simulink model "Final_Project_v3b"  (R2013a)
settings: Solver=ode45  StartTime=0.0  StopTime=inf  RelTol=1e-3
InitFcn:
  | start_EEVSCube2
  | 
  | %links masses
  | 
  | m=20;%Kg
  | 
  | l=1;%meter
  | 
  | %controls
  | 
  | a=0.3; %singularity positive gain
  | 
  | %Chaser
  | 
  | lb=1;%meter distance 1joint to CM
  | 
  | %Target
  | 
  | mt=5;%kg target mass
  | lt=1;%meter  side lenght
  | It=(1/6)*(lt^2);
  | 
  | %Target Initial Conitions
  | 
  | x_t=2;
  | y_t=3;
  | theta_t=0.7853;
  | 
  | Init_t=[x_t;y_t;theta_t];
undefined symbols (not defined in the file or in its folder): mesh_A, mesh_B
libraries: vrlib x2, dspinverses x1, aerolibanimutils x1
(part 2 of 2)

== matlab function Final_Project_v3b/Torque Control/C Matrix ==
  data: qqd input; C output; m parameter; l parameter; q_dot output
function [C,q_dot] = fcn(qqd,m,l)
q=[qqd(7); qqd(8); qqd(9)];
q_dot=[qqd(4); qqd(5); qqd(6)];
C=[                                                                                                                                                                                                                                                                                                                                                                                                                                                                                                                                                  (m*abs(l)^2*(2*sin(conj(q(1))) + sin(conj(q(1)) + conj(q(2)) + conj(q(3))) + 2*sin(conj(q(1)) + conj(q(2))))*(cos(q(1) + q(2) + q(3))*(q_dot(1) + q_dot(2) + q_dot(3)) + 2*cos(q(1) + q(2))*(q_dot(1) + q_dot(2)) + 2*q_dot(1)*cos(q(1))))/8 - (m*abs(l)^2*(2*cos(conj(q(1))) + cos(conj(q(1)) + conj(q(2)) + conj(q(3))) + 2*cos(conj(q(1)) + conj(q(2))))*(sin(q(1) + q(2) + q(3))*(q_dot(1) + q_dot(2) + q_dot(3)) + 2*sin(q(1) + q(2))*(q_dot(1) + q_dot(2)) + 2*q_dot(1)*sin(q(1))))/8 + (m*abs(l)^2*(cos(q(1) + q(2))*(q_dot(1) + q_dot(2)) + 2*q_dot(1)*cos(q(1)))*(2*sin(conj(q(1))) + sin(conj(q(1)) + conj(q(2)))))/8 - (m*abs(l)^2*(2*cos(conj(q(1))) + cos(conj(q(1)) + conj(q(2))))*(sin(q(1) + q(2))*(q_dot(1) + q_dot(2)) + 2*q_dot(1)*sin(q(1))))/8 - (m*abs(l)^2*(cos(q(1) + q(2)) + 2*cos(q(1)))*(2*sin(conj(q(1)))*conj(q_dot(1)) + sin(conj(q(1)) + conj(q(2)))*(conj(q_dot(1)) + conj(q_dot(2)))))/8 + (m*abs(l)^2*(sin(q(1) + q(2)) + 2*sin(q(1)))*(2*cos(conj(q(1)))*conj(q_dot(1)) + cos(conj(q(1)) + conj(q(2)))*(conj(q_dot(1)) + conj(q_dot(2)))))/8 + (m*abs(l)^2*(2*cos(conj(q(1)))*conj(q_dot(1)) + cos(conj(q(1)) + conj(q(2)) + conj(q(3)))*(conj(q_dot(1)) + conj(q_dot(2)) + conj(q_dot(3))) + 2*cos(conj(q(1)) + conj(q(2)))*(conj(q_dot(1)) + conj(q_dot(2))))*(sin(q(1) + q(2) + q(3)) + 2*sin(q(1) + q(2)) + 2*sin(q(1))))/8 - (m*abs(l)^2*(2*sin(conj(q(1)))*conj(q_dot(1)) + sin(conj(q(1)) + conj(q(2)) + conj(q(3)))*(conj(q_dot(1)) + conj(q_dot(2)) + conj(q_dot(3))) + 2*sin(conj(q(1)) + conj(q(2)))*(conj(q_dot(1)) + conj(q_dot(2))))*(cos(q(1) + q(2) + q(3)) + 2*cos(q(1) + q(2)) + 2*cos(q(1))))/8 - (m*q_dot(1)*cos(conj(q(1)))*abs(l)^2*sin(q(1)))/8 + (m*q_dot(1)*sin(conj(q(1)))*abs(l)^2*cos(q(1)))/8 + (m*cos(conj(q(1)))*abs(l)^2*conj(q_dot(1))*sin(q(1)))/8 - (m*sin(conj(q(1)))*abs(l)^2*cos(q(1))*conj(q_dot(1)))/8,                                                                                                                                                                                                                                     (m*sin(conj(q(1)) - q(2) - q(3) - q(1))*abs(l)^2)/2 + (3*m*sin(conj(q(1)) - q(2) - q(1))*abs(l)^2)/4 + (m*abs(l)^2*sin(conj(q(1)) - q(2) - q(3) - q(1) + conj(q(2)))*(q_dot(1) + q_dot(2) + q_dot(3) - conj(q_dot(1)) - conj(q_dot(2))))/4 + (m*sin(conj(q(1)) - q(2) - q(3) - q(1) + conj(q(2)) + conj(q(3)))*abs(l)^2*(q_dot(1) + q_dot(2) + q_dot(3) - conj(q_dot(1)) - conj(q_dot(2)) - conj(q_dot(3))))/8 - (m*sin(q(1) + q(2))*abs(l)^2*(2*cos(conj(q(1))) + cos(conj(q(1)) + conj(q(2)))))/8 + (m*cos(q(1) + q(2))*abs(l)^2*(2*sin(conj(q(1))) + sin(conj(q(1)) + conj(q(2)))))/8 - (m*abs(l)^2*(sin(conj(q(1)) + conj(q(2)) + conj(q(3))) + 2*sin(conj(q(1)) + conj(q(2))))*(cos(q(1) + q(2) + q(3)) + 2*cos(q(1) + q(2)) + 2*cos(q(1))))/8 + (m*abs(l)^2*(cos(conj(q(1)) + conj(q(2)) + conj(q(3))) + 2*cos(conj(q(1)) + conj(q(2))))*(sin(q(1) + q(2) + q(3)) + 2*sin(q(1) + q(2)) + 2*sin(q(1))))/8 - (m*abs(l)^2*sin(conj(q(1)) - q(2) - q(1) + conj(q(2)) + conj(q(3)))*(conj(q_dot(1)) - q_dot(2) - q_dot(1) + conj(q_dot(2)) + conj(q_dot(3))))/4 - (m*abs(l)^2*(sin(q(1) + q(2) + q(3)) + 2*sin(q(1) + q(2)))*(2*cos(conj(q(1))) + cos(conj(q(1)) + conj(q(2)) + conj(q(3))) + 2*cos(conj(q(1)) + conj(q(2)))))/8 + (m*abs(l)^2*(cos(q(1) + q(2) + q(3)) + 2*cos(q(1) + q(2)))*(2*sin(conj(q(1))) + sin(conj(q(1)) + conj(q(2)) + conj(q(3))) + 2*sin(conj(q(1)) + conj(q(2)))))/8 - (m*sin(conj(q(1)) + conj(q(2)))*abs(l)^2*(cos(q(1) + q(2)) + 2*cos(q(1))))/8 + (3*m*sin(conj(q(1)) - q(2) - q(1))*abs(l)^2*(q_dot(1) + q_dot(2) - conj(q_dot(1))))/4 + (m*cos(conj(q(1)) + conj(q(2)))*abs(l)^2*(sin(q(1) + q(2)) + 2*sin(q(1))))/8 + (5*m*sin(conj(q(1)) - q(2) - q(1) + conj(q(2)))*abs(l)^2*(q_dot(1) + q_dot(2) - conj(q_dot(1)) - conj(q_dot(2))))/8 + (m*sin(conj(q(1)) - q(2) - q(3) - q(1))*abs(l)^2*(q_dot(1) + q_dot(2) + q_dot(3) - conj(q_dot(1))))/4, (m*sin(conj(q(1)) - q(2) - q(3) - q(1))*abs(l)^2)/4 + (m*abs(l)^2*(2*sin(conj(q(1)) - q(2) - q(3) - q(1)) + 2*sin(conj(q(1)) - q(2) - q(3) - q(1) + conj(q(2)))))/8 + (m*abs(l)^2*(2*sin(conj(q(1)) - q(2) - q(3) - q(1))*(q_dot(1) + q_dot(2) + q_dot(3) - conj(q_dot(1))) + 2*sin(conj(q(1)) - q(2) - q(3) - q(1) + conj(q(2)))*(q_dot(1) + q_dot(2) + q_dot(3) - conj(q_dot(1)) - conj(q_dot(2))) + sin(conj(q(1)) - q(2) - q(3) - q(1) + conj(q(2)) + conj(q(3)))*(q_dot(1) + q_dot(2) + q_dot(3) - conj(q_dot(1)) - conj(q_dot(2)) - conj(q_dot(3)))))/8 + (m*abs(l)^2*sin(conj(q(1)) - q(2) - q(3) - q(1) + conj(q(2))))/4 - (m*abs(l)^2*sin(conj(q(1)) - q(2) - q(1) + conj(q(2)) + conj(q(3))))/4 + (m*cos(conj(q(1)) + conj(q(2)) + conj(q(3)))*abs(l)^2*(sin(q(1) + q(2) + q(3)) + 2*sin(q(1) + q(2)) + 2*sin(q(1))))/8 - (m*sin(q(1) + q(2) + q(3))*abs(l)^2*(2*cos(conj(q(1))) + cos(conj(q(1)) + conj(q(2)) + conj(q(3))) + 2*cos(conj(q(1)) + conj(q(2)))))/8 + (m*cos(q(1) + q(2) + q(3))*abs(l)^2*(2*sin(conj(q(1))) + sin(conj(q(1)) + conj(q(2)) + conj(q(3))) + 2*sin(conj(q(1)) + conj(q(2)))))/8 - (m*sin(conj(q(1)) + conj(q(2)) + conj(q(3)))*abs(l)^2*(cos(q(1) + q(2) + q(3)) + 2*cos(q(1) + q(2)) + 2*cos(q(1))))/8;
 (m*sin(conj(q(1)) - q(2) - q(3) - q(1))*abs(l)^2)/2 + (3*m*sin(conj(q(1)) - q(2) - q(1))*abs(l)^2)/4 - (m*abs(l)^2*(cos(conj(q(1)) + conj(q(2)) + conj(q(3))) + 2*cos(conj(q(1)) + conj(q(2))))*(sin(q(1) + q(2) + q(3))*(q_dot(1) + q_dot(2) + q_dot(3)) + 2*sin(q(1) + q(2))*(q_dot(1) + q_dot(2)) + 2*q_dot(1)*sin(q(1))))/8 - (m*sin(q(1) + q(2))*abs(l)^2*(2*cos(conj(q(1))) + cos(conj(q(1)) + conj(q(2)))))/8 + (m*cos(q(1) + q(2))*abs(l)^2*(2*sin(conj(q(1))) + sin(conj(q(1)) + conj(q(2)))))/8 - (m*abs(l)^2*(sin(conj(q(1)) + conj(q(2)) + conj(q(3))) + 2*sin(conj(q(1)) + conj(q(2))))*(cos(q(1) + q(2) + q(3)) + 2*cos(q(1) + q(2)) + 2*cos(q(1))))/8 + (m*abs(l)^2*(cos(conj(q(1)) + conj(q(2)) + conj(q(3))) + 2*cos(conj(q(1)) + conj(q(2))))*(sin(q(1) + q(2) + q(3)) + 2*sin(q(1) + q(2)) + 2*sin(q(1))))/8 - (m*abs(l)^2*(sin(conj(q(1)) + conj(q(2)) + conj(q(3)))*(conj(q_dot(1)) + conj(q_dot(2)) + conj(q_dot(3))) + 2*sin(conj(q(1)) + conj(q(2)))*(conj(q_dot(1)) + conj(q_dot(2))))*(cos(q(1) + q(2) + q(3)) + 2*cos(q(1) + q(2)) + 2*cos(q(1))))/8 + (m*abs(l)^2*(cos(conj(q(1)) + conj(q(2)) + conj(q(3)))*(conj(q_dot(1)) + conj(q_dot(2)) + conj(q_dot(3))) + 2*cos(conj(q(1)) + conj(q(2)))*(conj(q_dot(1)) + conj(q_dot(2))))*(sin(q(1) + q(2) + q(3)) + 2*sin(q(1) + q(2)) + 2*sin(q(1))))/8 - (m*abs(l)^2*(sin(q(1) + q(2) + q(3)) + 2*sin(q(1) + q(2)))*(2*cos(conj(q(1))) + cos(conj(q(1)) + conj(q(2)) + conj(q(3))) + 2*cos(conj(q(1)) + conj(q(2)))))/8 + (m*abs(l)^2*(cos(q(1) + q(2) + q(3)) + 2*cos(q(1) + q(2)))*(2*sin(conj(q(1))) + sin(conj(q(1)) + conj(q(2)) + conj(q(3))) + 2*sin(conj(q(1)) + conj(q(2)))))/8 - (m*sin(conj(q(1)) + conj(q(2)))*abs(l)^2*(cos(q(1) + q(2)) + 2*cos(q(1))))/8 + (m*cos(conj(q(1)) + conj(q(2)))*abs(l)^2*(sin(q(1) + q(2)) + 2*sin(q(1))))/8 + (m*sin(conj(q(1)) + conj(q(2)))*abs(l)^2*(cos(q(1) + q(2))*(q_dot(1) + q_dot(2)) + 2*q_dot(1)*cos(q(1))))/8 - (m*cos(conj(q(1)) + conj(q(2)))*abs(l)^2*(sin(q(1) + q(2))*(q_dot(1) + q_dot(2)) + 2*q_dot(1)*sin(q(1))))/8 + (m*abs(l)^2*(sin(conj(q(1)) + conj(q(2)) + conj(q(3))) + 2*sin(conj(q(1)) + conj(q(2))))*(cos(q(1) + q(2) + q(3))*(q_dot(1) + q_dot(2) + q_dot(3)) + 2*cos(q(1) + q(2))*(q_dot(1) + q_dot(2)) + 2*q_dot(1)*cos(q(1))))/8 - (m*sin(conj(q(1)) + conj(q(2)))*abs(l)^2*(conj(q_dot(1)) + conj(q_dot(2)))*(cos(q(1) + q(2)) + 2*cos(q(1))))/8 + (m*cos(conj(q(1)) + conj(q(2)))*abs(l)^2*(conj(q_dot(1)) + conj(q_dot(2)))*(sin(q(1) + q(2)) + 2*sin(q(1))))/8, (m*sin(conj(q(1)) + conj(q(2)))*cos(q(1) + q(2))*abs(l)^2)/4 - (m*cos(conj(q(1)) + conj(q(2)))*sin(q(1) + q(2))*abs(l)^2)/4 - (m*abs(l)^2*(sin(conj(q(1)) + conj(q(2)) + conj(q(3))) + 2*sin(conj(q(1)) + conj(q(2))))*(cos(q(1) + q(2) + q(3)) + 2*cos(q(1) + q(2)) + 2*cos(q(1))))/4 + (m*abs(l)^2*(cos(conj(q(1)) + conj(q(2)) + conj(q(3))) + 2*cos(conj(q(1)) + conj(q(2))))*(sin(q(1) + q(2) + q(3)) + 2*sin(q(1) + q(2)) + 2*sin(q(1))))/4 - (m*abs(l)^2*(cos(q(1) + q(2) + q(3)) + 2*cos(q(1) + q(2)))*(sin(conj(q(1)) + conj(q(2)) + conj(q(3)))*(conj(q_dot(1)) + conj(q_dot(2)) + conj(q_dot(3))) + 2*sin(conj(q(1)) + conj(q(2)))*(conj(q_dot(1)) + conj(q_dot(2)))))/8 + (m*abs(l)^2*(sin(q(1) + q(2) + q(3)) + 2*sin(q(1) + q(2)))*(cos(conj(q(1)) + conj(q(2)) + conj(q(3)))*(conj(q_dot(1)) + conj(q_dot(2)) + conj(q_dot(3))) + 2*cos(conj(q(1)) + conj(q(2)))*(conj(q_dot(1)) + conj(q_dot(2)))))/8 - (m*abs(l)^2*(cos(conj(q(1)) + conj(q(2)) + conj(q(3))) + 2*cos(conj(q(1)) + conj(q(2))))*(sin(q(1) + q(2) + q(3))*(q_dot(1) + q_dot(2) + q_dot(3)) + 2*sin(q(1) + q(2))*(q_dot(1) + q_dot(2))))/8 + (m*abs(l)^2*(sin(conj(q(1)) + conj(q(2)) + conj(q(3))) + 2*sin(conj(q(1)) + conj(q(2))))*(cos(q(1) + q(2) + q(3))*(q_dot(1) + q_dot(2) + q_dot(3)) + 2*cos(q(1) + q(2))*(q_dot(1) + q_dot(2))))/8 - (m*sin(conj(q(1)) + conj(q(2)))*abs(l)^2*(cos(q(1) + q(2)) + 2*cos(q(1))))/4 + (m*cos(conj(q(1)) + conj(q(2)))*abs(l)^2*(sin(q(1) + q(2)) + 2*sin(q(1))))/4 - (m*abs(l)^2*(cos(conj(q(1)) + conj(q(2)) + conj(q(3))) + 2*cos(conj(q(1)) + conj(q(2))))*(sin(q(1) + q(2) + q(3)) + 2*sin(q(1) + q(2))))/4 + (m*abs(l)^2*(cos(q(1) + q(2) + q(3)) + 2*cos(q(1) + q(2)))*(sin(conj(q(1)) + conj(q(2)) + conj(q(3))) + 2*sin(conj(q(1)) + conj(q(2)))))/4 + (m*cos(conj(q(1)) + conj(q(2)))*sin(q(1) + q(2))*abs(l)^2*(conj(q_dot(1)) + conj(q_dot(2))))/8 - (m*sin(conj(q(1)) + conj(q(2)))*cos(q(1) + q(2))*abs(l)^2*(conj(q_dot(1)) + conj(q_dot(2))))/8 - (m*cos(conj(q(1)) + conj(q(2)))*sin(q(1) + q(2))*abs(l)^2*(q_dot(1) + q_dot(2)))/8 + (m*sin(conj(q(1)) + conj(q(2)))*cos(q(1) + q(2))*abs(l)^2*(q_dot(1) + q_dot(2)))/8,                                                                                                                                                                                                                                                                                                                       (m*abs(l)^2*(2*sin(conj(q(1)) - q(2) - q(3) - q(1) + conj(q(2)))*(q_dot(1) + q_dot(2) + q_dot(3) - conj(q_dot(1)) - conj(q_dot(2))) + sin(conj(q(1)) - q(2) - q(3) - q(1) + conj(q(2)) + conj(q(3)))*(q_dot(1) + q_dot(2) + q_dot(3) - conj(q_dot(1)) - conj(q_dot(2)) - conj(q_dot(3)))))/8 + (m*abs(l)^2*sin(conj(q(1)) - q(2) - q(3) - q(1) + conj(q(2))))/4 + (m*cos(conj(q(1)) + conj(q(2)) + conj(q(3)))*abs(l)^2*(sin(q(1) + q(2) + q(3)) + 2*sin(q(1) + q(2)) + 2*sin(q(1))))/4 - (m*sin(q(1) + q(2) + q(3))*abs(l)^2*(cos(conj(q(1)) + conj(q(2)) + conj(q(3))) + 2*cos(conj(q(1)) + conj(q(2)))))/4 + (m*cos(q(1) + q(2) + q(3))*abs(l)^2*(sin(conj(q(1)) + conj(q(2)) + conj(q(3))) + 2*sin(conj(q(1)) + conj(q(2)))))/4 - (m*sin(conj(q(1)) + conj(q(2)) + conj(q(3)))*abs(l)^2*(cos(q(1) + q(2) + q(3)) + 2*cos(q(1) + q(2)) + 2*cos(q(1))))/4;
                                                                                                                                                                                                                                                                                                                                                                                                                                                                                                                                                                                                                                                                                                                                                                                                      (m*sin(conj(q(1)) - q(2) - q(3) - q(1))*abs(l)^2)/4 + (m*abs(l)^2*(2*sin(conj(q(1)) - q(2) - q(3) - q(1)) + 2*sin(conj(q(1)) - q(2) - q(3) - q(1) + conj(q(2)))))/8 + (m*abs(l)^2*sin(conj(q(1)) - q(2) - q(3) - q(1) + conj(q(2))))/4 - (m*abs(l)^2*sin(conj(q(1)) - q(2) - q(1) + conj(q(2)) + conj(q(3))))/4 + (m*cos(conj(q(1)) + conj(q(2)) + conj(q(3)))*abs(l)^2*(sin(q(1) + q(2) + q(3)) + 2*sin(q(1) + q(2)) + 2*sin(q(1))))/8 - (m*sin(q(1) + q(2) + q(3))*abs(l)^2*(2*cos(conj(q(1))) + cos(conj(q(1)) + conj(q(2)) + conj(q(3))) + 2*cos(conj(q(1)) + conj(q(2)))))/8 + (m*cos(q(1) + q(2) + q(3))*abs(l)^2*(2*sin(conj(q(1))) + sin(conj(q(1)) + conj(q(2)) + conj(q(3))) + 2*sin(conj(q(1)) + conj(q(2)))))/8 + (m*sin(conj(q(1)) + conj(q(2)) + conj(q(3)))*abs(l)^2*(cos(q(1) + q(2) + q(3))*(q_dot(1) + q_dot(2) + q_dot(3)) + 2*cos(q(1) + q(2))*(q_dot(1) + q_dot(2)) + 2*q_dot(1)*cos(q(1))))/8 - (m*cos(conj(q(1)) + conj(q(2)) + conj(q(3)))*abs(l)^2*(sin(q(1) + q(2) + q(3))*(q_dot(1) + q_dot(2) + q_dot(3)) + 2*sin(q(1) + q(2))*(q_dot(1) + q_dot(2)) + 2*q_dot(1)*sin(q(1))))/8 - (m*sin(conj(q(1)) + conj(q(2)) + conj(q(3)))*abs(l)^2*(cos(q(1) + q(2) + q(3)) + 2*cos(q(1) + q(2)) + 2*cos(q(1))))/8 - (m*sin(conj(q(1)) + conj(q(2)) + conj(q(3)))*abs(l)^2*(cos(q(1) + q(2) + q(3)) + 2*cos(q(1) + q(2)) + 2*cos(q(1)))*(conj(q_dot(1)) + conj(q_dot(2)) + conj(q_dot(3))))/8 + (m*cos(conj(q(1)) + conj(q(2)) + conj(q(3)))*abs(l)^2*(sin(q(1) + q(2) + q(3)) + 2*sin(q(1) + q(2)) + 2*sin(q(1)))*(conj(q_dot(1)) + conj(q_dot(2)) + conj(q_dot(3))))/8,                                                                                                                                                                                                                                                                                                                                                                                                                                                                                                                                                                                                                                                                                                                                                                                                            (m*abs(l)^2*sin(conj(q(1)) - q(2) - q(3) - q(1) + conj(q(2))))/4 + (m*cos(conj(q(1)) + conj(q(2)) + conj(q(3)))*abs(l)^2*(sin(q(1) + q(2) + q(3)) + 2*sin(q(1) + q(2)) + 2*sin(q(1))))/4 + (m*sin(conj(q(1)) + conj(q(2)) + conj(q(3)))*abs(l)^2*(cos(q(1) + q(2) + q(3))*(q_dot(1) + q_dot(2) + q_dot(3)) + 2*cos(q(1) + q(2))*(q_dot(1) + q_dot(2))))/8 - (m*cos(conj(q(1)) + conj(q(2)) + conj(q(3)))*abs(l)^2*(sin(q(1) + q(2) + q(3))*(q_dot(1) + q_dot(2) + q_dot(3)) + 2*sin(q(1) + q(2))*(q_dot(1) + q_dot(2))))/8 - (m*sin(q(1) + q(2) + q(3))*abs(l)^2*(cos(conj(q(1)) + conj(q(2)) + conj(q(3))) + 2*cos(conj(q(1)) + conj(q(2)))))/4 + (m*cos(q(1) + q(2) + q(3))*abs(l)^2*(sin(conj(q(1)) + conj(q(2)) + conj(q(3))) + 2*sin(conj(q(1)) + conj(q(2)))))/4 - (m*sin(conj(q(1)) + conj(q(2)) + conj(q(3)))*abs(l)^2*(cos(q(1) + q(2) + q(3)) + 2*cos(q(1) + q(2)) + 2*cos(q(1))))/4 - (m*sin(conj(q(1)) + conj(q(2)) + conj(q(3)))*abs(l)^2*(cos(q(1) + q(2) + q(3)) + 2*cos(q(1) + q(2)))*(conj(q_dot(1)) + conj(q_dot(2)) + conj(q_dot(3))))/8 + (m*cos(conj(q(1)) + conj(q(2)) + conj(q(3)))*abs(l)^2*(sin(q(1) + q(2) + q(3)) + 2*sin(q(1) + q(2)))*(conj(q_dot(1)) + conj(q_dot(2)) + conj(q_dot(3))))/8,                                                                                                                                                                                                                                                                                                                                                            (m*sin(conj(q(1)) - q(2) - q(3) - q(1) + conj(q(2)) + conj(q(3)))*abs(l)^2*(q_dot(1) + q_dot(2) + q_dot(3) - conj(q_dot(1)) - conj(q_dot(2)) - conj(q_dot(3))))/8 + (m*cos(conj(q(1)) + conj(q(2)) + conj(q(3)))*abs(l)^2*(sin(q(1) + q(2) + q(3)) + 2*sin(q(1) + q(2)) + 2*sin(q(1))))/4 + (m*cos(q(1) + q(2) + q(3))*sin(conj(q(1)) + conj(q(2)) + conj(q(3)))*abs(l)^2)/2 - (m*sin(q(1) + q(2) + q(3))*cos(conj(q(1)) + conj(q(2)) + conj(q(3)))*abs(l)^2)/2 - (m*sin(conj(q(1)) + conj(q(2)) + conj(q(3)))*abs(l)^2*(cos(q(1) + q(2) + q(3)) + 2*cos(q(1) + q(2))))/4 + (m*cos(conj(q(1)) + conj(q(2)) + conj(q(3)))*abs(l)^2*(sin(q(1) + q(2) + q(3)) + 2*sin(q(1) + q(2))))/4 - (m*sin(conj(q(1)) + conj(q(2)) + conj(q(3)))*abs(l)^2*(cos(q(1) + q(2) + q(3)) + 2*cos(q(1) + q(2)) + 2*cos(q(1))))/4];

== matlab function Final_Project_v3b/Torque Control/G Matrix (set zero) ==
  data: qqd input; G output; l parameter; m parameter
function G = fcn(qqd,l,m)

q=[qqd(7); qqd(8); qqd(9)];

g=[0 9.81 0]; %gravity acceleration along y


Jp1=[-(l/2)*sin(q(1)) 0 0; (l/2)*cos(q(1)) 0 0; 0 0 0];
Jo1=[0 0 0; 0 0 0; 1 0 0];

Jp2=[-l*sin(q(1))-(l/2)*sin(q(1)+q(2)) -(l/2)*sin(q(1)+q(2)) 0 ;    l*cos(q(1))+(l/2)*cos(q(1)+q(2)) (l/2)*cos(q(1)+q(2)) 0; 0 0 0];
Jo2=[0 0 0; 0 0 0; 1 1 0];

Jp3=[-l*sin(q(1))-l*sin(q(1)+q(2))-(l/2)*sin(q(1)+q(2)+q(3)) -l*sin(q(1)+q(2))-(l/2)*sin(q(1)+q(2)+q(3)) -(l/2)*sin(q(1)+q(2)+q(3)); l*cos(q(1))+(l)*cos(q(1)+q(2))+(l/2)*cos(q(1)+q(2)+q(3)) l*cos(q(1)+q(2))+(l/2)*cos(q(1)+q(2)+q(3)) (l/2)*cos(q(1)+q(2)+q(3)); 0 0 0];
Jo3=[0 0 0; 0 0 0; 1 1 1];

G1=m*(g)*Jp1+m*(g)*Jp2+m*(g)*Jp3;

%G=G1.';

G=[0;0;0];

== matlab function Final_Project_v3b/Torque Control/H Matrix ==
  data: H output; qqd input; l parameter; m parameter
function H = fcn(qqd,l,m)

q=[qqd(7); qqd(8); qqd(9)];
I=(1/12)*m*(l^2); 
%Hand derivation of the Jacobians for the three links
Jp1=[-(l/2)*sin(q(1)) 0 0; (l/2)*cos(q(1)) 0 0; 0 0 0];
Jo1=[0 0 0; 0 0 0; 1 0 0];

Jp2=[-l*sin(q(1))-(l/2)*sin(q(1)+q(2)) -(l/2)*sin(q(1)+q(2)) 0 ;    l*cos(q(1))+(l/2)*cos(q(1)+q(2)) (l/2)*cos(q(1)+q(2)) 0; 0 0 0];
Jo2=[0 0 0; 0 0 0; 1 1 0];

Jp3=[-l*sin(q(1))-l*sin(q(1)+q(2))-(l/2)*sin(q(1)+q(2)+q(3)) -l*sin(q(1)+q(2))-(l/2)*sin(q(1)+q(2)+q(3)) -(l/2)*sin(q(1)+q(2)+q(3)); l*cos(q(1))+(l)*cos(q(1)+q(2))+(l/2)*cos(q(1)+q(2)+q(3)) l*cos(q(1)+q(2))+(l/2)*cos(q(1)+q(2)+q(3)) (l/2)*cos(q(1)+q(2)+q(3)); 0 0 0];
Jo3=[0 0 0; 0 0 0; 1 1 1];

%%%%%%%%%%%%%%%%%%%%%%%%%%%%%%%%%%%%%%%%%%%%%%%%%%%%%%%%%%%%%%%%%%%%%%%%%
% %Inertia Matrix H
H1=(m*(Jp1')*Jp1)+(Jo1'*I*Jo1); %should be Hermitian? ???????????    
H2=(m*(Jp2')*Jp2)+(Jo2'*I*Jo2);
H3=(m*(Jp3')*Jp3)+(Jo3'*I*Jo3);
%Total Inertia Matrix
H=H1+H2+H3;

== matlab function Final_Project_v3b/Dynamics Block/H Matrix ==
  data: H output; qqd input; l parameter; m parameter
function H = fcn(qqd,l,m)

q=[qqd(7) qqd(8) qqd(9)];
I=(1/12)*m*(l^2); 
%Hand derivation of the Jacobians for the three links
Jp1=[-(l/2)*sin(q(1)) 0 0; (l/2)*cos(q(1)) 0 0; 0 0 0];
Jo1=[0 0 0; 0 0 0; 1 0 0];

Jp2=[-l*sin(q(1))-(l/2)*sin(q(1)+q(2)) -(l/2)*sin(q(1)+q(2)) 0 ;    l*cos(q(1))+(l/2)*cos(q(1)+q(2)) (l/2)*cos(q(1)+q(2)) 0; 0 0 0];
Jo2=[0 0 0; 0 0 0; 1 1 0];

Jp3=[-l*sin(q(1))-l*sin(q(1)+q(2))-(l/2)*sin(q(1)+q(2)+q(3)) -l*sin(q(1)+q(2))-(l/2)*sin(q(1)+q(2)+q(3)) -(l/2)*sin(q(1)+q(2)+q(3)); l*cos(q(1))+(l)*cos(q(1)+q(2))+(l/2)*cos(q(1)+q(2)+q(3)) l*cos(q(1)+q(2))+(l/2)*cos(q(1)+q(2)+q(3)) (l/2)*cos(q(1)+q(2)+q(3)); 0 0 0];
Jo3=[0 0 0; 0 0 0; 1 1 1];

%%%%%%%%%%%%%%%%%%%%%%%%%%%%%%%%%%%%%%%%%%%%%%%%%%%%%%%%%%%%%%%%%%%%%%%%%
% %Inertia Matrix H
H1=(m*(Jp1')*Jp1)+(Jo1'*I*Jo1); %should be Hermitian? ???????????    
H2=(m*(Jp2')*Jp2)+(Jo2'*I*Jo2);
H3=(m*(Jp3')*Jp3)+(Jo3'*I*Jo3);
%Total Inertia Matrix
H=H1+H2+H3;

== matlab function Final_Project_v3b/Singularity Check ==
  data: qqd input; Ya output; l parameter
function Ya   = fcn( qqd,l)
%Singularity trigger, Alessio Grompone 2013

q=[qqd(7) qqd(8) qqd(9)];

%if A==0
%Jacobian position only

Ja=[-(l*sin(q(1))+l*sin(q(1)+q(2))+l*sin(q(1)+q(2)+q(3))) -(l*sin(q(1)+q(2))+l*sin(q(1)+q(2)+q(3))) -l*sin(q(1)+q(2)+q(3));
l*cos(q(1))+l*cos(q(1)+q(2))+l*cos(q(1)+q(2)+q(3)) l*cos(q(1)+q(2))+l*cos(q(1)+q(2)+q(3)) l*cos(q(1)+q(2)+q(3))];

Ra=rank(Ja); %rank of the Jacobian
Sa=size(Ja); %dimension of the Jacobian matrix

if Ra<Sa(1)

Ya=0; %non singular

else
    
Ya=1;
    
end

== matlab function Final_Project_v3b/Differential Kinematics/Differential Kinematics and singularity avoidance ==
  data: Ve input; qqd input; qd_req output; qd_reqW output; l parameter; a parameter; W output; EE input
function [qd_req,qd_reqW,W]   = fcn( Ve,qqd, l, a,EE)
%Singularity trigger, Alessio Grompone 2013

%computes the Jacobian of a redundant 3R manipulator (end-effector position
%only)measures the rank and gives an error if the rank is < than the number of
%variables

q=[qqd(7) qqd(8) qqd(9)];

%Jacobian position only

Ja=[-(l*sin(q(1))+l*sin(q(1)+q(2))+l*sin(q(1)+q(2)+q(3))) -(l*sin(q(1)+q(2))+l*sin(q(1)+q(2)+q(3))) -l*sin(q(1)+q(2)+q(3));
l*cos(q(1))+l*cos(q(1)+q(2))+l*cos(q(1)+q(2)+q(3)) l*cos(q(1)+q(2))+l*cos(q(1)+q(2)+q(3)) l*cos(q(1)+q(2)+q(3))];

DDD=det(Ja*Ja');
%     %Singularity Measure
% 
W=sqrt(DDD);
if q(2)==0
    
    DW=[0;0;0];
else
%Derivative of the singularity measure obtained in symbolic form
    DW=[                                                                                                                                                                                                                                                                                                                                                                                                                                                                                                                                                                                                                                                                                                                                                                                                                                                                                                                                                                                                                                                                                                                                                                                                                                                                                                                                                                                                                                                                                                                                                                                                                                                                                                                                                                                                                                                                                                                                                                                                                                                                                                                                                                                                                                                                                                                                                                                                                                                                                                                                                                                                                                                                                                                                                                                                                                                                                                                                                                                                                                                                                                                                                                                                                                                                                                                                                                                                                                                                                                                                                                                                                                                                                                                                                                                                                                                                                                                                                                                                                                                                                                                                                                                                                                                                                                                                                                                                                                                                                                                                                                                                                                                                                                                                                                                                                                                                                                                                                                                                                                                                                                                                                                                                                                                                                                                                                                                                                                                                                                                                                                                                                                                                                                                                                                                  0;
                                                                                                                                                                                                                                                                                                                                                                                                                 -(cos(q(1) + q(2) + q(3))*cos(conj(q(1)) + conj(q(2)) + conj(q(3)))*sin(conj(q(1)) + conj(q(2)))*cos(q(1)) - cos(q(1) + q(2) + q(3))*sin(conj(q(1)) + conj(q(2)) + conj(q(3)))*cos(conj(q(1)) + conj(q(2)))*cos(q(1)) + cos(q(1) + q(2) + q(3))*sin(conj(q(1)))*sin(conj(q(1)) + conj(q(2)))*sin(q(1)) - sin(q(1) + q(2) + q(3))*cos(conj(q(1)))*sin(conj(q(1)) + conj(q(2)))*sin(q(1)) + sin(q(1) + q(2) + q(3))*sin(conj(q(1)))*cos(conj(q(1)) + conj(q(2)))*sin(q(1)) - sin(q(1) + q(2) + q(3))*sin(conj(q(1)))*sin(conj(q(1)) + conj(q(2)))*cos(q(1)) + sin(q(1) + q(2) + q(3))*cos(conj(q(1)) + conj(q(2)) + conj(q(3)))*sin(conj(q(1)) + conj(q(2)))*sin(q(1)) - sin(q(1) + q(2) + q(3))*sin(conj(q(1)) + conj(q(2)) + conj(q(3)))*cos(conj(q(1)) + conj(q(2)))*sin(q(1)) + cos(conj(q(1)))*cos(conj(q(1)) + conj(q(2)) + conj(q(3)))*cos(q(1) + q(2))*sin(q(1)) - cos(conj(q(1)))*cos(conj(q(1)) + conj(q(2)) + conj(q(3)))*sin(q(1) + q(2))*cos(q(1)) - cos(conj(q(1)))*sin(conj(q(1)) + conj(q(2)) + conj(q(3)))*cos(q(1) + q(2))*cos(q(1)) + cos(conj(q(1)) + conj(q(2)) + conj(q(3)))*sin(conj(q(1)))*cos(q(1) + q(2))*cos(q(1)) - cos(conj(q(1)))*sin(conj(q(1)) + conj(q(2)) + conj(q(3)))*sin(q(1) + q(2))*sin(q(1)) + cos(conj(q(1)) + conj(q(2)) + conj(q(3)))*sin(conj(q(1)))*sin(q(1) + q(2))*sin(q(1)) + sin(conj(q(1)))*sin(conj(q(1)) + conj(q(2)) + conj(q(3)))*cos(q(1) + q(2))*sin(q(1)) - sin(conj(q(1)))*sin(conj(q(1)) + conj(q(2)) + conj(q(3)))*sin(q(1) + q(2))*cos(q(1)) + cos(conj(q(1)))*cos(conj(q(1)) + conj(q(2)))*cos(q(1) + q(2))*sin(q(1)) - cos(conj(q(1)))*cos(conj(q(1)) + conj(q(2)))*sin(q(1) + q(2))*cos(q(1)) - cos(conj(q(1)))*sin(conj(q(1)) + conj(q(2)))*cos(q(1) + q(2))*cos(q(1)) + sin(conj(q(1)))*cos(conj(q(1)) + conj(q(2)))*cos(q(1) + q(2))*cos(q(1)) + cos(q(1) + q(2) + q(3))*cos(conj(q(1)))*cos(conj(q(1)) + conj(q(2)) + conj(q(3)))*sin(q(1) + q(2)) - sin(q(1) + q(2) + q(3))*cos(conj(q(1)))*cos(conj(q(1)) + conj(q(2)) + conj(q(3)))*cos(q(1) + q(2)) - cos(conj(q(1)))*sin(conj(q(1)) + conj(q(2)))*sin(q(1) + q(2))*sin(q(1)) + sin(conj(q(1)))*cos(conj(q(1)) + conj(q(2)))*sin(q(1) + q(2))*sin(q(1)) + sin(conj(q(1)))*sin(conj(q(1)) + conj(q(2)))*cos(q(1) + q(2))*sin(q(1)) - sin(conj(q(1)))*sin(conj(q(1)) + conj(q(2)))*sin(q(1) + q(2))*cos(q(1)) + cos(q(1) + q(2) + q(3))*sin(conj(q(1)))*sin(conj(q(1)) + conj(q(2)) + conj(q(3)))*sin(q(1) + q(2)) - sin(q(1) + q(2) + q(3))*sin(conj(q(1)))*sin(conj(q(1)) + conj(q(2)) + conj(q(3)))*cos(q(1) + q(2)) + 2*cos(q(1) + q(2) + q(3))*cos(conj(q(1)))*cos(conj(q(1)) + conj(q(2)) + conj(q(3)))*sin(q(1)) - 2*cos(q(1) + q(2) + q(3))*cos(conj(q(1)))*sin(conj(q(1)) + conj(q(2)) + conj(q(3)))*cos(q(1)) + 2*cos(q(1) + q(2) + q(3))*cos(conj(q(1)) + conj(q(2)) + conj(q(3)))*sin(conj(q(1)))*cos(q(1)) - 2*sin(q(1) + q(2) + q(3))*cos(conj(q(1)))*cos(conj(q(1)) + conj(q(2)) + conj(q(3)))*cos(q(1)) + 2*cos(q(1) + q(2) + q(3))*sin(conj(q(1)))*sin(conj(q(1)) + conj(q(2)) + conj(q(3)))*sin(q(1)) - 2*sin(q(1) + q(2) + q(3))*cos(conj(q(1)))*sin(conj(q(1)) + conj(q(2)) + conj(q(3)))*sin(q(1)) + 2*sin(q(1) + q(2) + q(3))*cos(conj(q(1)) + conj(q(2)) + conj(q(3)))*sin(conj(q(1)))*sin(q(1)) - 2*sin(q(1) + q(2) + q(3))*sin(conj(q(1)))*sin(conj(q(1)) + conj(q(2)) + conj(q(3)))*cos(q(1)) + cos(q(1) + q(2) + q(3))*cos(conj(q(1)))*cos(conj(q(1)) + conj(q(2)))*sin(q(1)) - cos(q(1) + q(2) + q(3))*cos(conj(q(1)))*sin(conj(q(1)) + conj(q(2)))*cos(q(1)) + cos(q(1) + q(2) + q(3))*sin(conj(q(1)))*cos(conj(q(1)) + conj(q(2)))*cos(q(1)) - sin(q(1) + q(2) + q(3))*cos(conj(q(1)))*cos(conj(q(1)) + conj(q(2)))*cos(q(1)))/(2*(cos(q(1) + q(2) + q(3))*sin(conj(q(1)))*cos(conj(q(1)) + conj(q(2)))*sin(q(1)) - cos(q(1) + q(2) + q(3))*cos(conj(q(1)))*sin(conj(q(1)) + conj(q(2)))*sin(q(1)) + sin(q(1) + q(2) + q(3))*cos(conj(q(1)))*sin(conj(q(1)) + conj(q(2)))*cos(q(1)) - sin(q(1) + q(2) + q(3))*sin(conj(q(1)))*cos(conj(q(1)) + conj(q(2)))*cos(q(1)) + cos(q(1) + q(2) + q(3))*cos(conj(q(1)) + conj(q(2)) + conj(q(3)))*sin(conj(q(1)) + conj(q(2)))*sin(q(1)) - cos(q(1) + q(2) + q(3))*sin(conj(q(1)) + conj(q(2)) + conj(q(3)))*cos(conj(q(1)) + conj(q(2)))*sin(q(1)) - sin(q(1) + q(2) + q(3))*cos(conj(q(1)) + conj(q(2)) + conj(q(3)))*sin(conj(q(1)) + conj(q(2)))*cos(q(1)) + sin(q(1) + q(2) + q(3))*sin(conj(q(1)) + conj(q(2)) + conj(q(3)))*cos(conj(q(1)) + conj(q(2)))*cos(q(1)) - cos(conj(q(1)))*sin(conj(q(1)) + conj(q(2)) + conj(q(3)))*cos(q(1) + q(2))*sin(q(1)) + cos(conj(q(1)))*sin(conj(q(1)) + conj(q(2)) + conj(q(3)))*sin(q(1) + q(2))*cos(q(1)) + cos(conj(q(1)) + conj(q(2)) + conj(q(3)))*sin(conj(q(1)))*cos(q(1) + q(2))*sin(q(1)) - cos(conj(q(1)) + conj(q(2)) + conj(q(3)))*sin(conj(q(1)))*sin(q(1) + q(2))*cos(q(1)) - cos(conj(q(1)))*sin(conj(q(1)) + conj(q(2)))*cos(q(1) + q(2))*sin(q(1)) + cos(conj(q(1)))*sin(conj(q(1)) + conj(q(2)))*sin(q(1) + q(2))*cos(q(1)) + sin(conj(q(1)))*cos(conj(q(1)) + conj(q(2)))*cos(q(1) + q(2))*sin(q(1)) - sin(conj(q(1)))*cos(conj(q(1)) + conj(q(2)))*sin(q(1) + q(2))*cos(q(1)) - cos(q(1) + q(2) + q(3))*cos(conj(q(1)))*sin(conj(q(1)) + conj(q(2)) + conj(q(3)))*sin(q(1) + q(2)) + cos(q(1) + q(2) + q(3))*cos(conj(q(1)) + conj(q(2)) + conj(q(3)))*sin(conj(q(1)))*sin(q(1) + q(2)) + sin(q(1) + q(2) + q(3))*cos(conj(q(1)))*sin(conj(q(1)) + conj(q(2)) + conj(q(3)))*cos(q(1) + q(2)) - sin(q(1) + q(2) + q(3))*cos(conj(q(1)) + conj(q(2)) + conj(q(3)))*sin(conj(q(1)))*cos(q(1) + q(2)) - 2*cos(q(1) + q(2) + q(3))*cos(conj(q(1)))*sin(conj(q(1)) + conj(q(2)) + conj(q(3)))*sin(q(1)) + 2*cos(q(1) + q(2) + q(3))*cos(conj(q(1)) + conj(q(2)) + conj(q(3)))*sin(conj(q(1)))*sin(q(1)) + 2*sin(q(1) + q(2) + q(3))*cos(conj(q(1)))*sin(conj(q(1)) + conj(q(2)) + conj(q(3)))*cos(q(1)) - 2*sin(q(1) + q(2) + q(3))*cos(conj(q(1)) + conj(q(2)) + conj(q(3)))*sin(conj(q(1)))*cos(q(1)) + 2*cos(q(1) + q(2) + q(3))*cos(conj(q(1)) + conj(q(2)) + conj(q(3)))*sin(conj(q(1)) + conj(q(2)))*sin(q(1) + q(2)) - 2*cos(q(1) + q(2) + q(3))*sin(conj(q(1)) + conj(q(2)) + conj(q(3)))*cos(conj(q(1)) + conj(q(2)))*sin(q(1) + q(2)) - 2*sin(q(1) + q(2) + q(3))*cos(conj(q(1)) + conj(q(2)) + conj(q(3)))*sin(conj(q(1)) + conj(q(2)))*cos(q(1) + q(2)) + 2*sin(q(1) + q(2) + q(3))*sin(conj(q(1)) + conj(q(2)) + conj(q(3)))*cos(conj(q(1)) + conj(q(2)))*cos(q(1) + q(2)))^(1/2));
 -(cos(q(1) + q(2) + q(3))*cos(conj(q(1)) + conj(q(2)) + conj(q(3)))*cos(conj(q(1)) + conj(q(2)))*sin(q(1)) + cos(q(1) + q(2) + q(3))*cos(conj(q(1)) + conj(q(2)) + conj(q(3)))*sin(conj(q(1)) + conj(q(2)))*cos(q(1)) - cos(q(1) + q(2) + q(3))*sin(conj(q(1)) + conj(q(2)) + conj(q(3)))*cos(conj(q(1)) + conj(q(2)))*cos(q(1)) - sin(q(1) + q(2) + q(3))*cos(conj(q(1)) + conj(q(2)) + conj(q(3)))*cos(conj(q(1)) + conj(q(2)))*cos(q(1)) - sin(q(1) + q(2) + q(3))*cos(conj(q(1)))*sin(conj(q(1)) + conj(q(2)))*sin(q(1)) + sin(q(1) + q(2) + q(3))*sin(conj(q(1)))*cos(conj(q(1)) + conj(q(2)))*sin(q(1)) + cos(q(1) + q(2) + q(3))*sin(conj(q(1)) + conj(q(2)) + conj(q(3)))*sin(conj(q(1)) + conj(q(2)))*sin(q(1)) + sin(q(1) + q(2) + q(3))*cos(conj(q(1)) + conj(q(2)) + conj(q(3)))*sin(conj(q(1)) + conj(q(2)))*sin(q(1)) - sin(q(1) + q(2) + q(3))*sin(conj(q(1)) + conj(q(2)) + conj(q(3)))*cos(conj(q(1)) + conj(q(2)))*sin(q(1)) - sin(q(1) + q(2) + q(3))*sin(conj(q(1)) + conj(q(2)) + conj(q(3)))*sin(conj(q(1)) + conj(q(2)))*cos(q(1)) + cos(conj(q(1)))*cos(conj(q(1)) + conj(q(2)) + conj(q(3)))*cos(q(1) + q(2))*sin(q(1)) - cos(conj(q(1)))*cos(conj(q(1)) + conj(q(2)) + conj(q(3)))*sin(q(1) + q(2))*cos(q(1)) + sin(conj(q(1)))*sin(conj(q(1)) + conj(q(2)) + conj(q(3)))*cos(q(1) + q(2))*sin(q(1)) - sin(conj(q(1)))*sin(conj(q(1)) + conj(q(2)) + conj(q(3)))*sin(q(1) + q(2))*cos(q(1)) + cos(q(1) + q(2) + q(3))*cos(conj(q(1)))*cos(conj(q(1)) + conj(q(2)) + conj(q(3)))*sin(q(1) + q(2)) - cos(q(1) + q(2) + q(3))*cos(conj(q(1)))*sin(conj(q(1)) + conj(q(2)) + conj(q(3)))*cos(q(1) + q(2)) + cos(q(1) + q(2) + q(3))*cos(conj(q(1)) + conj(q(2)) + conj(q(3)))*sin(conj(q(1)))*cos(q(1) + q(2)) - sin(q(1) + q(2) + q(3))*cos(conj(q(1)))*cos(conj(q(1)) + conj(q(2)) + conj(q(3)))*cos(q(1) + q(2)) + cos(q(1) + q(2) + q(3))*sin(conj(q(1)))*sin(conj(q(1)) + conj(q(2)) + conj(q(3)))*sin(q(1) + q(2)) - sin(q(1) + q(2) + q(3))*cos(conj(q(1)))*sin(conj(q(1)) + conj(q(2)) + conj(q(3)))*sin(q(1) + q(2)) + sin(q(1) + q(2) + q(3))*cos(conj(q(1)) + conj(q(2)) + conj(q(3)))*sin(conj(q(1)))*sin(q(1) + q(2)) - sin(q(1) + q(2) + q(3))*sin(conj(q(1)))*sin(conj(q(1)) + conj(q(2)) + conj(q(3)))*cos(q(1) + q(2)) + 2*cos(q(1) + q(2) + q(3))*cos(conj(q(1)))*cos(conj(q(1)) + conj(q(2)) + conj(q(3)))*sin(q(1)) - 2*cos(q(1) + q(2) + q(3))*cos(conj(q(1)))*sin(conj(q(1)) + conj(q(2)) + conj(q(3)))*cos(q(1)) + 2*cos(q(1) + q(2) + q(3))*cos(conj(q(1)) + conj(q(2)) + conj(q(3)))*sin(conj(q(1)))*cos(q(1)) - 2*sin(q(1) + q(2) + q(3))*cos(conj(q(1)))*cos(conj(q(1)) + conj(q(2)) + conj(q(3)))*cos(q(1)) + 2*cos(q(1) + q(2) + q(3))*cos(conj(q(1)) + conj(q(2)) + conj(q(3)))*cos(conj(q(1)) + conj(q(2)))*sin(q(1) + q(2)) + 2*cos(q(1) + q(2) + q(3))*cos(conj(q(1)) + conj(q(2)) + conj(q(3)))*sin(conj(q(1)) + conj(q(2)))*cos(q(1) + q(2)) - 2*cos(q(1) + q(2) + q(3))*sin(conj(q(1)) + conj(q(2)) + conj(q(3)))*cos(conj(q(1)) + conj(q(2)))*cos(q(1) + q(2)) - 2*sin(q(1) + q(2) + q(3))*cos(conj(q(1)) + conj(q(2)) + conj(q(3)))*cos(conj(q(1)) + conj(q(2)))*cos(q(1) + q(2)) + 2*cos(q(1) + q(2) + q(3))*sin(conj(q(1)))*sin(conj(q(1)) + conj(q(2)) + conj(q(3)))*sin(q(1)) - 2*sin(q(1) + q(2) + q(3))*cos(conj(q(1)))*sin(conj(q(1)) + conj(q(2)) + conj(q(3)))*sin(q(1)) + 2*sin(q(1) + q(2) + q(3))*cos(conj(q(1)) + conj(q(2)) + conj(q(3)))*sin(conj(q(1)))*sin(q(1)) - 2*sin(q(1) + q(2) + q(3))*sin(conj(q(1)))*sin(conj(q(1)) + conj(q(2)) + conj(q(3)))*cos(q(1)) + 2*cos(q(1) + q(2) + q(3))*sin(conj(q(1)) + conj(q(2)) + conj(q(3)))*sin(conj(q(1)) + conj(q(2)))*sin(q(1) + q(2)) + 2*sin(q(1) + q(2) + q(3))*cos(conj(q(1)) + conj(q(2)) + conj(q(3)))*sin(conj(q(1)) + conj(q(2)))*sin(q(1) + q(2)) - 2*sin(q(1) + q(2) + q(3))*sin(conj(q(1)) + conj(q(2)) + conj(q(3)))*cos(conj(q(1)) + conj(q(2)))*sin(q(1) + q(2)) - 2*sin(q(1) + q(2) + q(3))*sin(conj(q(1)) + conj(q(2)) + conj(q(3)))*sin(conj(q(1)) + conj(q(2)))*cos(q(1) + q(2)) - cos(q(1) + q(2) + q(3))*cos(conj(q(1)))*sin(conj(q(1)) + conj(q(2)))*cos(q(1)) + cos(q(1) + q(2) + q(3))*sin(conj(q(1)))*cos(conj(q(1)) + conj(q(2)))*cos(q(1)))/(2*(cos(q(1) + q(2) + q(3))*sin(conj(q(1)))*cos(conj(q(1)) + conj(q(2)))*sin(q(1)) - cos(q(1) + q(2) + q(3))*cos(conj(q(1)))*sin(conj(q(1)) + conj(q(2)))*sin(q(1)) + sin(q(1) + q(2) + q(3))*cos(conj(q(1)))*sin(conj(q(1)) + conj(q(2)))*cos(q(1)) - sin(q(1) + q(2) + q(3))*sin(conj(q(1)))*cos(conj(q(1)) + conj(q(2)))*cos(q(1)) + cos(q(1) + q(2) + q(3))*cos(conj(q(1)) + conj(q(2)) + conj(q(3)))*sin(conj(q(1)) + conj(q(2)))*sin(q(1)) - cos(q(1) + q(2) + q(3))*sin(conj(q(1)) + conj(q(2)) + conj(q(3)))*cos(conj(q(1)) + conj(q(2)))*sin(q(1)) - sin(q(1) + q(2) + q(3))*cos(conj(q(1)) + conj(q(2)) + conj(q(3)))*sin(conj(q(1)) + conj(q(2)))*cos(q(1)) + sin(q(1) + q(2) + q(3))*sin(conj(q(1)) + conj(q(2)) + conj(q(3)))*cos(conj(q(1)) + conj(q(2)))*cos(q(1)) - cos(conj(q(1)))*sin(conj(q(1)) + conj(q(2)) + conj(q(3)))*cos(q(1) + q(2))*sin(q(1)) + cos(conj(q(1)))*sin(conj(q(1)) + conj(q(2)) + conj(q(3)))*sin(q(1) + q(2))*cos(q(1)) + cos(conj(q(1)) + conj(q(2)) + conj(q(3)))*sin(conj(q(1)))*cos(q(1) + q(2))*sin(q(1)) - cos(conj(q(1)) + conj(q(2)) + conj(q(3)))*sin(conj(q(1)))*sin(q(1) + q(2))*cos(q(1)) - cos(conj(q(1)))*sin(conj(q(1)) + conj(q(2)))*cos(q(1) + q(2))*sin(q(1)) + cos(conj(q(1)))*sin(conj(q(1)) + conj(q(2)))*sin(q(1) + q(2))*cos(q(1)) + sin(conj(q(1)))*cos(conj(q(1)) + conj(q(2)))*cos(q(1) + q(2))*sin(q(1)) - sin(conj(q(1)))*cos(conj(q(1)) + conj(q(2)))*sin(q(1) + q(2))*cos(q(1)) - cos(q(1) + q(2) + q(3))*cos(conj(q(1)))*sin(conj(q(1)) + conj(q(2)) + conj(q(3)))*sin(q(1) + q(2)) + cos(q(1) + q(2) + q(3))*cos(conj(q(1)) + conj(q(2)) + conj(q(3)))*sin(conj(q(1)))*sin(q(1) + q(2)) + sin(q(1) + q(2) + q(3))*cos(conj(q(1)))*sin(conj(q(1)) + conj(q(2)) + conj(q(3)))*cos(q(1) + q(2)) - sin(q(1) + q(2) + q(3))*cos(conj(q(1)) + conj(q(2)) + conj(q(3)))*sin(conj(q(1)))*cos(q(1) + q(2)) - 2*cos(q(1) + q(2) + q(3))*cos(conj(q(1)))*sin(conj(q(1)) + conj(q(2)) + conj(q(3)))*sin(q(1)) + 2*cos(q(1) + q(2) + q(3))*cos(conj(q(1)) + conj(q(2)) + conj(q(3)))*sin(conj(q(1)))*sin(q(1)) + 2*sin(q(1) + q(2) + q(3))*cos(conj(q(1)))*sin(conj(q(1)) + conj(q(2)) + conj(q(3)))*cos(q(1)) - 2*sin(q(1) + q(2) + q(3))*cos(conj(q(1)) + conj(q(2)) + conj(q(3)))*sin(conj(q(1)))*cos(q(1)) + 2*cos(q(1) + q(2) + q(3))*cos(conj(q(1)) + conj(q(2)) + conj(q(3)))*sin(conj(q(1)) + conj(q(2)))*sin(q(1) + q(2)) - 2*cos(q(1) + q(2) + q(3))*sin(conj(q(1)) + conj(q(2)) + conj(q(3)))*cos(conj(q(1)) + conj(q(2)))*sin(q(1) + q(2)) - 2*sin(q(1) + q(2) + q(3))*cos(conj(q(1)) + conj(q(2)) + conj(q(3)))*sin(conj(q(1)) + conj(q(2)))*cos(q(1) + q(2)) + 2*sin(q(1) + q(2) + q(3))*sin(conj(q(1)) + conj(q(2)) + conj(q(3)))*cos(conj(q(1)) + conj(q(2)))*cos(q(1) + q(2)))^(1/2))];
end
Jstar=pinv(Ja); %inverse of the Jacobian

qa=a*DW;

qd_req=Jstar*Ve;
qd_reqW=Jstar*Ve+(eye(3)-Jstar*Ja)*qa;%With singularity avoidance

qd_req(3)=qd_req(3)+EE;
qd_reqW(3)=qd_reqW(3)+EE;
end

== matlab function Final_Project_v3b/GamePad Input/MATLAB Function ==
  data: u output; but output; Axes input; Buttons input; j output
function [u,but,j]  = fcn(Axes,Buttons)
%#Mapping buttons for KRAUN Gamepad
%Alessio Grompone

%%%%%%%%%%%%%%%%%%%%%%%%%%%%%%%%%%%%%%%%%%%%%%%%%%%%
%       Home Gamepad
%Axes

if Axes(2)==-1
    %Up
    u=[1;0];
elseif Axes(2)==1
        %Down
    u=[-1;0];   
elseif  Axes(1)==-1
    %Left
    u=[0;1];
elseif  Axes(1)==1 
    %Right
    u=[0;-1];
else
    %NO Axes Command
    u=[0;0];
end

if Buttons(5)==1
j=1;
else
if Buttons(6)==1
    j=-1;
else
    j=0;
end
end

if Buttons(1)==1
    %Button1
    but=[0;0;0;0];
elseif Buttons(1)==1
    %Button1
    but=[0;0;0;0];
elseif Buttons(1)==1
    %Button1
    but=[0;0;0;0];
elseif Buttons(1)==1
    %Button1
    but=[0;0;0;0];
else
    %NO Button command
    but=[0;0;0;0];
end
end

== matlab function Final_Project_v3b/Collision/Collision/Collision ==
  data: epsilon input; dock_sensA_c output; dock_sensB_c output; n_c output; QA_c output; QB_c output; sigma_dock input; dotsigma_dock input; Rbi_A1 input; Rbi_B1 input; A output; B output; Xcm_A input; Xcm_B input; mesh_A input; mesh_B input; dock_sensA input; dock_sensB input; sigma input; docking output; ma_mb_Ia_Ib input; collision output; Vcm_an output; Vcm_bn output; W_an output; W_bn output; j output
function [dock_sensA_c,dock_sensB_c,n_c,QA_c,QB_c,A,B,docking,collision,Vcm_an,Vcm_bn,W_an,W_bn,j] = fcn(epsilon,sigma_dock,dotsigma_dock,Rbi_A1,Rbi_B1,Xcm_A,Xcm_B,mesh_A,mesh_B,dock_sensA,dock_sensB,sigma,ma_mb_Ia_Ib)

[dock_sensA_c,dock_sensB_c,n_c,QA_c,QB_c,A,B,docking,collision,Vcm_an,Vcm_bn,W_an,W_bn,j] = collision_function(epsilon,sigma_dock,dotsigma_dock,Rbi_A1,Rbi_B1,Xcm_A,Xcm_B,mesh_A,mesh_B,dock_sensA,dock_sensB,sigma,ma_mb_Ia_Ib);

== matlab function Final_Project_v3b/Collision/Collision/Embedded MATLAB Function10 ==
  data: M input; DD output
function DD=fcn(M)

[m,n] = size(M);
a = zeros(n*m,1);
MM=zeros(n*m,1);
i=1;
for mm=0:m:n*m-1
for j=1:1:m
    a(j+mm,1)=M(j,i); 
end
i=i+1;
end
DD=a;

== matlab function Final_Project_v3b/Collision/Collision/Embedded MATLAB Function9 ==
  data: M input; DD output
function DD=fcn(M)

[m,n] = size(M);
a = zeros(n*m,1);
MM=zeros(n*m,1);
i=1;
for mm=0:m:n*m-1
for j=1:1:m
    a(j+mm,1)=M(j,i); 
end
i=i+1;
end
DD=a;

== matlab function Final_Project_v3b/Collision/StateVectormapping2/Target State Vector ==
  data: u1 input; y output; u2 input; u3 input; u4 input; u5 input; u6 input; collision input; memory input
function y  = fcn(u1,u2,u3,u4,u5,u6,collision,memory)
%#codegen


if collision==1

y=[u1;u2;u3;u4;u5;u6];

else
    
y=[u1;u2;u3;memory(4);memory(5);memory(6)];

end

== matlab function Final_Project_v3b/Collision/StateVectormapping/Rotation MAtrix1 ==
  data: u input; y output; R output
function [y,R] = fcn(u)
%#codegen

y=[u(1);u(2); 0; u(4); u(5); 0; 0; 0; u(6)];



R = [cos(u(3)) -sin(u(3));
    sin(u(3)) cos(u(3))];

end

== matlab function Final_Project_v3b/3rd link Kinematics ==
  data: qqd input; state_3link output; lb parameter; l parameter
function state_3link = fcn(qqd,lb,l)
%#codegen

%fixed base position

xb=0;
yb=0;
thetab=0;
thetabb=0;

state_3link=zeros([6,1]);

state_3link(1)=lb*cos(thetab)+l*cos(qqd(7)+thetab)+l*cos(qqd(8)+qqd(7)+thetab)+(l/2)*cos(qqd(9)+qqd(8)+qqd(7)+thetab);%X inertia position of the CM of the third Link
state_3link(2)=lb*sin(thetab)+l*sin(qqd(7)+thetab)+l*sin(qqd(8)+qqd(7)+thetab)+(l/2)*sin(qqd(9)+qqd(8)+qqd(7)+thetab);%Y inertia position of the CM of the third Link
state_3link(3)=qqd(9)+qqd(8)+qqd(7)+thetab;%theta inertia position of the CM of the third Link
state_3link(4)=-lb*thetabb*sin(thetab)-l*(qqd(4)+thetabb)*sin(qqd(7)+thetab)-l*(qqd(4)+qqd(5)+thetabb)*sin(qqd(8)+qqd(7)+thetab)-(l/2)*(qqd(4)+qqd(5)+qqd(6)+thetabb)*sin(qqd(9)+qqd(8)+qqd(7)+thetab);%VX inertia position of the CM of the third Link
state_3link(5)=lb*thetabb*cos(thetab)+l*(qqd(4)+thetabb)*cos(qqd(7)+thetab)+l*(qqd(4)+qqd(5)+thetabb)*cos(qqd(8)+qqd(7)+thetab)+(l/2)*(qqd(4)+qqd(5)+qqd(6)+thetabb)*cos(qqd(9)+qqd(8)+qqd(7)+thetab);%VY inertia position of the CM of the third Link;%X inertia position of the CM of the third Link
state_3link(6)=qqd(4)+qqd(5)+qqd(6)+thetabb;%omega inertia position of the CM of the third Link

end

== matlab function Final_Project_v3b/Collision/StateVectormapping1/Rotation MAtrix1 ==
  data: u1 input; y output; R output; u2 input; u3 input; u4 input; u5 input; u6 input
function [y,R] = fcn(u1,u2,u3,u4,u5,u6)
%#codegen

% y=[u(1);u(2); 0; u(4); u(5); 0; 0; u(6)];

y=[u1;u2;0;u4;u5;0;0;0;u6];
theta=u3;

R = [cos(theta) -sin(theta);
    sin(theta) cos(theta)];

end
